simulink model "basic_model"  (R2024b)
settings: Solver=VariableStepAuto  StartTime=0.0  StopTime=0.4  FixedStep=5e-8  RelTol=1e-3

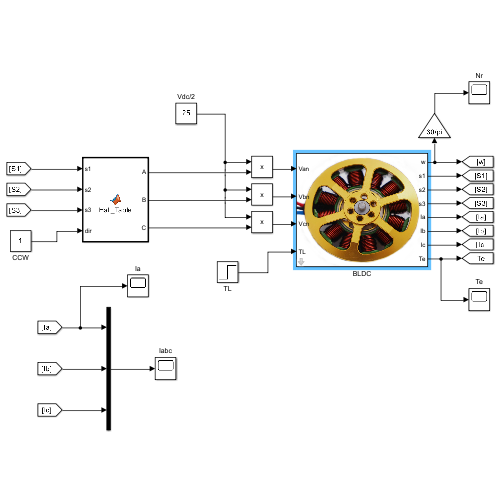
[thumbnail: Simulink's stored preview of the top-level diagram]
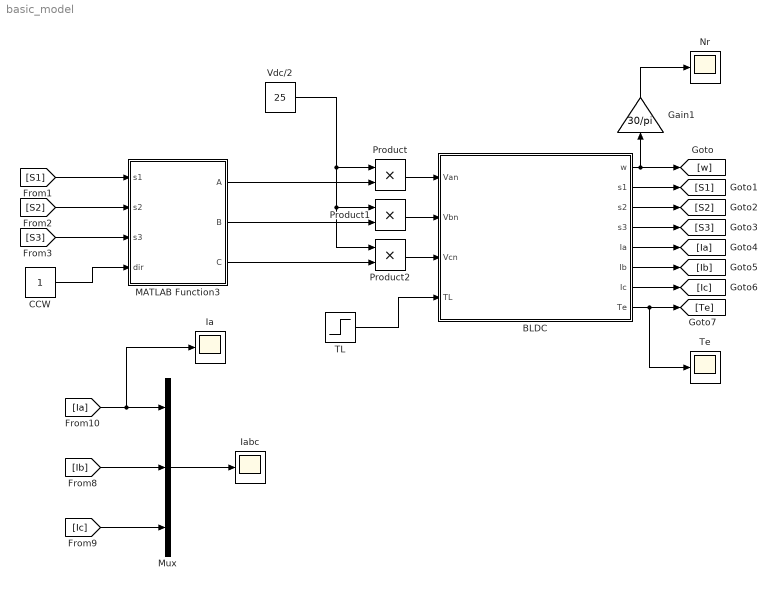
== system basic_model ==
  BLDC : Subsystem  mask(Function Block Parameters: BLDC){R=0.106/2, L=(0.428e-3)/2, b=0.0001, J=4.943e-4, Kt=0.164, Ke=0.164, pn=2}
      mask prompts: R "Phase Resistance"; L "Phase Inductance"; b "Viscous damping"; J "Rotor inertia"; Kt "Torque Sensitivity"; Ke "Back-EMF gain"; pn "poles pairs"
  CCW : Constant
  Gain1 : Gain  Gain=30/pi
  Ia : Scope
  Iabc : Scope
  MATLAB Function3 : MATLAB Function  TreatAsAtomicUnit=on
  Mux : Mux  Inputs=3
  Nr : Scope
  Product : Product
  Product1 : Product
  Product2 : Product
  TL : Step  Time=0.2  After=10  SampleTime=0
  Te : Scope
  Vdc/2 : Constant  Value=25
  wires:
  Vdc/2/1 -> Product2/1, Product1/1, Product/1
  BLDC/1(w) -> Gain1/1, [w]
  BLDC/2(s1) -> [S1]
  BLDC/3(s2) -> [S2]
  BLDC/4(s3) -> [S3]
  BLDC/5(Ia) -> [Ia]
  BLDC/6(Ib) -> [Ib]
  BLDC/7(Ic) -> [Ic]
  TL/1 -> BLDC/4(TL)
  [Ic] -> Mux/3
  [Ib] -> Mux/2
  [Ia] -> Ia/1, Mux/1
  MATLAB Function3/1(A) -> Product/2
  MATLAB Function3/2(B) -> Product1/2
  MATLAB Function3/3(C) -> Product2/2
  [S2] -> MATLAB Function3/2(s2)
  [S3] -> MATLAB Function3/3(s3)
  [S1] -> MATLAB Function3/1(s1)
  CCW/1 -> MATLAB Function3/4(dir)
  Gain1/1 -> Nr/1
  BLDC/8(Te) -> Te/1, [Te]
  Mux/1 -> Iabc/1
  Product2/1 -> BLDC/3(Vcn)
  Product/1 -> BLDC/1(Van)
  Product1/1 -> BLDC/2(Vbn)

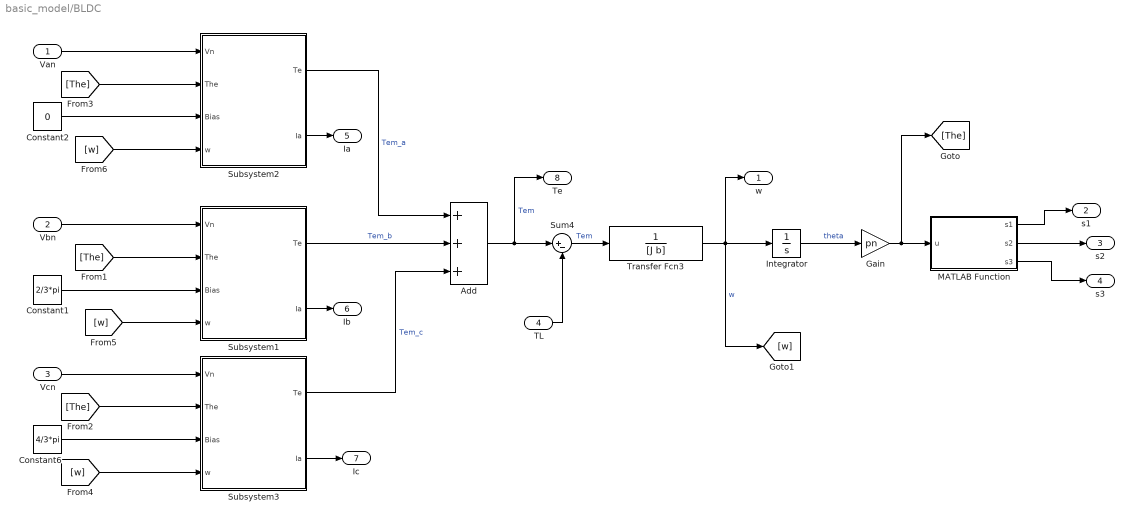
== system basic_model/BLDC ==
  Van : Inport
  Vbn : Inport  Port=2
  Vcn : Inport  Port=3
  TL : Inport  Port=4
  Add : Sum  Inputs=+++
  Constant1 : Constant  Value=2/3*pi
  Constant2 : Constant  Value=0
  Constant6 : Constant  Value=4/3*pi
  Gain : Gain  Gain=pn
  Integrator : Integrator
  MATLAB Function : MATLAB Function  TreatAsAtomicUnit=on
  Subsystem1 : Subsystem
  Subsystem2 : Subsystem
  Subsystem3 : Subsystem
  Sum4 : Sum  Inputs=|+-
  Transfer Fcn3 : TransferFcn  Denominator=[J b]
  w : Outport
  s1 : Outport  Port=2
  s2 : Outport  Port=3
  s3 : Outport  Port=4
  Ia : Outport  Port=5
  Ib : Outport  Port=6
  Ic : Outport  Port=7
  Te : Outport  Port=8
  wires:
  Vcn/1 -> Subsystem3/1(Vn)
  Sum4/1 -> Transfer Fcn3/1  "Tem"
  TL/1 -> Sum4/2
  Add/1 -> Te/1, Sum4/1  "Tem"
  Integrator/1 -> Gain/1  "theta"
  Transfer Fcn3/1 -> w/1, [w], Integrator/1  "w"
  [The] -> Subsystem3/2(The)
  Constant6/1 -> Subsystem3/3(Bias)
  Subsystem3/1(Te) -> Add/3  "Tem_c"
  Vbn/1 -> Subsystem1/1(Vn)
  Constant1/1 -> Subsystem1/3(Bias)
  [The] -> Subsystem1/2(The)
  Subsystem1/1(Te) -> Add/2  "Tem_b"
  Van/1 -> Subsystem2/1(Vn)
  Constant2/1 -> Subsystem2/3(Bias)
  [The] -> Subsystem2/2(The)
  Subsystem2/1(Te) -> Add/1  "Tem_a"
  [w] -> Subsystem3/4(w)
  [w] -> Subsystem1/4(w)
  [w] -> Subsystem2/4(w)
  Subsystem3/2(Ia) -> Ic/1
  Subsystem2/2(Ia) -> Ia/1
  MATLAB Function/1(s1) -> s1/1
  MATLAB Function/2(s2) -> s2/1
  MATLAB Function/3(s3) -> s3/1
  Subsystem1/2(Ia) -> Ib/1
  Gain/1 -> [The], MATLAB Function/1(u)

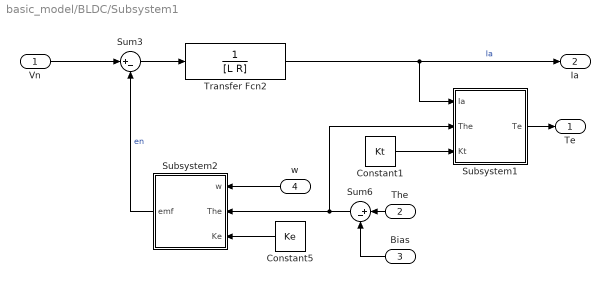
== system basic_model/BLDC/Subsystem1 ==
  Vn : Inport
  The : Inport  Port=2
  Bias : Inport  Port=3
  w : Inport  Port=4
  Constant1 : Constant  Value=Kt
  Constant5 : Constant  Value=Ke
  Subsystem1 : Subsystem
  Subsystem2 : Subsystem
  Sum3 : Sum  Inputs=|+-
  Sum6 : Sum  Inputs=|+-
  Transfer Fcn2 : TransferFcn  Denominator=[L R]
  Te : Outport
  Ia : Outport  Port=2
  wires:
  Bias/1 -> Sum6/2
  Subsystem2/1(emf) -> Sum3/2  "en"
  Sum6/1 -> Subsystem1/2(The), Subsystem2/2(The)
  Constant5/1 -> Subsystem2/3(Ke)
  w/1 -> Subsystem2/1(w)
  The/1 -> Sum6/1
  Constant1/1 -> Subsystem1/3(Kt)
  Subsystem1/1(Te) -> Te/1
  Sum3/1 -> Transfer Fcn2/1
  Vn/1 -> Sum3/1
  Transfer Fcn2/1 -> Subsystem1/1(Ia), Ia/1  "Ia"

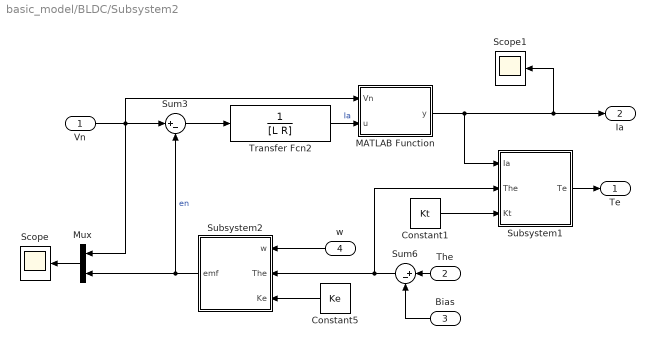
== system basic_model/BLDC/Subsystem2 ==
  Vn : Inport
  The : Inport  Port=2
  Bias : Inport  Port=3
  w : Inport  Port=4
  Constant1 : Constant  Value=Kt
  Constant5 : Constant  Value=Ke
  MATLAB Function : MATLAB Function  TreatAsAtomicUnit=on
  Mux : Mux  Inputs=2
  Scope : Scope
  Scope1 : Scope
  Subsystem1 : Subsystem
  Subsystem2 : Subsystem
  Sum3 : Sum  Inputs=|+-
  Sum6 : Sum  Inputs=|+-
  Transfer Fcn2 : TransferFcn  Denominator=[L R]
  Te : Outport
  Ia : Outport  Port=2
  wires:
  Bias/1 -> Sum6/2
  Subsystem2/1(emf) -> Sum3/2, Mux/2  "en"
  Sum6/1 -> Subsystem1/2(The), Subsystem2/2(The)
  Constant5/1 -> Subsystem2/3(Ke)
  w/1 -> Subsystem2/1(w)
  The/1 -> Sum6/1
  Constant1/1 -> Subsystem1/3(Kt)
  Subsystem1/1(Te) -> Te/1
  Mux/1 -> Scope/1
  Sum3/1 -> Transfer Fcn2/1
  Vn/1 -> Sum3/1, MATLAB Function/1(Vn), Mux/1
  Transfer Fcn2/1 -> MATLAB Function/2(u)  "Ia"
  MATLAB Function/1(y) -> Subsystem1/1(Ia), Scope1/1, Ia/1

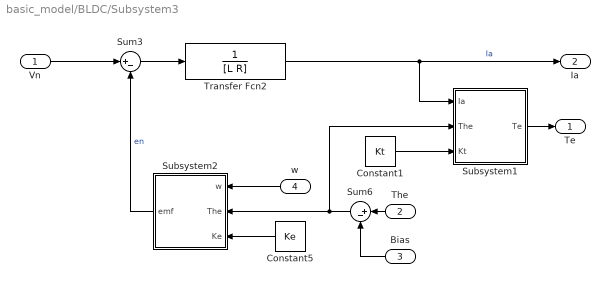
== system basic_model/BLDC/Subsystem3 ==
  Vn : Inport
  The : Inport  Port=2
  Bias : Inport  Port=3
  w : Inport  Port=4
  Constant1 : Constant  Value=Kt
  Constant5 : Constant  Value=Ke
  Subsystem1 : Subsystem
  Subsystem2 : Subsystem
  Sum3 : Sum  Inputs=|+-
  Sum6 : Sum  Inputs=|+-
  Transfer Fcn2 : TransferFcn  Denominator=[L R]
  Te : Outport
  Ia : Outport  Port=2
  wires:
  Bias/1 -> Sum6/2
  Subsystem2/1(emf) -> Sum3/2  "en"
  Sum6/1 -> Subsystem1/2(The), Subsystem2/2(The)
  Constant5/1 -> Subsystem2/3(Ke)
  w/1 -> Subsystem2/1(w)
  The/1 -> Sum6/1
  Constant1/1 -> Subsystem1/3(Kt)
  Subsystem1/1(Te) -> Te/1
  Sum3/1 -> Transfer Fcn2/1
  Vn/1 -> Sum3/1
  Transfer Fcn2/1 -> Subsystem1/1(Ia), Ia/1  "Ia"

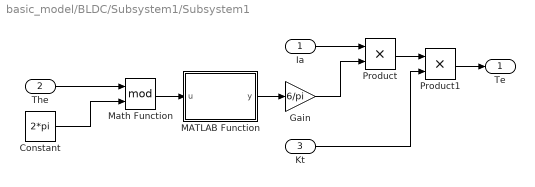
== system basic_model/BLDC/Subsystem1/Subsystem1 ==
  Ia : Inport
  The : Inport  Port=2
  Kt : Inport  Port=3
  Constant : Constant  Value=2*pi
  Gain : Gain  Gain=6/pi
  MATLAB Function : MATLAB Function  TreatAsAtomicUnit=on
  Math Function : Math  Operator=mod
  Product : Product
  Product1 : Product
  Te : Outport
  wires:
  The/1 -> Math Function/1
  Constant/1 -> Math Function/2
  Math Function/1 -> MATLAB Function/1(u)
  MATLAB Function/1(y) -> Gain/1
  Ia/1 -> Product/1
  Gain/1 -> Product/2
  Product/1 -> Product1/1
  Kt/1 -> Product1/2
  Product1/1 -> Te/1

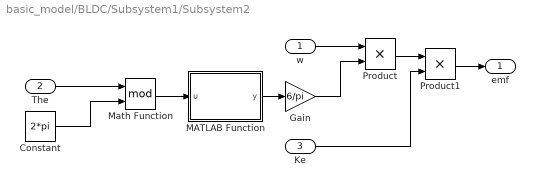
== system basic_model/BLDC/Subsystem1/Subsystem2 ==
  w : Inport
  The : Inport  Port=2
  Ke : Inport  Port=3
  Constant : Constant  Value=2*pi
  Gain : Gain  Gain=6/pi
  MATLAB Function : MATLAB Function  TreatAsAtomicUnit=on
  Math Function : Math  Operator=mod
  Product : Product
  Product1 : Product
  emf : Outport
  wires:
  The/1 -> Math Function/1
  Constant/1 -> Math Function/2
  Math Function/1 -> MATLAB Function/1(u)
  MATLAB Function/1(y) -> Gain/1
  w/1 -> Product/1
  Gain/1 -> Product/2
  Product/1 -> Product1/1
  Ke/1 -> Product1/2
  Product1/1 -> emf/1

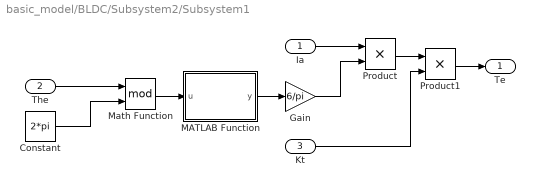
== system basic_model/BLDC/Subsystem2/Subsystem1 ==
  Ia : Inport
  The : Inport  Port=2
  Kt : Inport  Port=3
  Constant : Constant  Value=2*pi
  Gain : Gain  Gain=6/pi
  MATLAB Function : MATLAB Function  TreatAsAtomicUnit=on
  Math Function : Math  Operator=mod
  Product : Product
  Product1 : Product
  Te : Outport
  wires:
  The/1 -> Math Function/1
  Constant/1 -> Math Function/2
  Math Function/1 -> MATLAB Function/1(u)
  MATLAB Function/1(y) -> Gain/1
  Ia/1 -> Product/1
  Gain/1 -> Product/2
  Product/1 -> Product1/1
  Kt/1 -> Product1/2
  Product1/1 -> Te/1

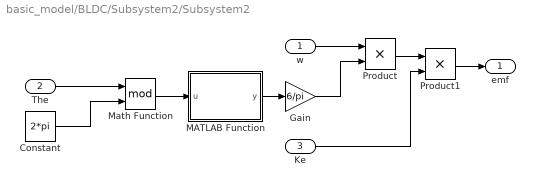
== system basic_model/BLDC/Subsystem2/Subsystem2 ==
  w : Inport
  The : Inport  Port=2
  Ke : Inport  Port=3
  Constant : Constant  Value=2*pi
  Gain : Gain  Gain=6/pi
  MATLAB Function : MATLAB Function  TreatAsAtomicUnit=on
  Math Function : Math  Operator=mod
  Product : Product
  Product1 : Product
  emf : Outport
  wires:
  The/1 -> Math Function/1
  Constant/1 -> Math Function/2
  Math Function/1 -> MATLAB Function/1(u)
  MATLAB Function/1(y) -> Gain/1
  w/1 -> Product/1
  Gain/1 -> Product/2
  Product/1 -> Product1/1
  Ke/1 -> Product1/2
  Product1/1 -> emf/1

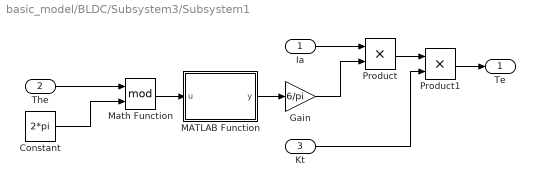
== system basic_model/BLDC/Subsystem3/Subsystem1 ==
  Ia : Inport
  The : Inport  Port=2
  Kt : Inport  Port=3
  Constant : Constant  Value=2*pi
  Gain : Gain  Gain=6/pi
  MATLAB Function : MATLAB Function  TreatAsAtomicUnit=on
  Math Function : Math  Operator=mod
  Product : Product
  Product1 : Product
  Te : Outport
  wires:
  The/1 -> Math Function/1
  Constant/1 -> Math Function/2
  Math Function/1 -> MATLAB Function/1(u)
  MATLAB Function/1(y) -> Gain/1
  Ia/1 -> Product/1
  Gain/1 -> Product/2
  Product/1 -> Product1/1
  Kt/1 -> Product1/2
  Product1/1 -> Te/1

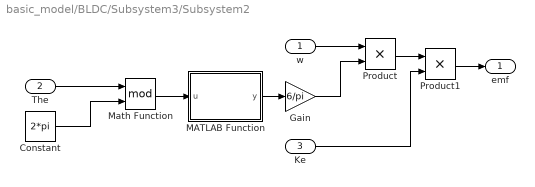
== system basic_model/BLDC/Subsystem3/Subsystem2 ==
  w : Inport
  The : Inport  Port=2
  Ke : Inport  Port=3
  Constant : Constant  Value=2*pi
  Gain : Gain  Gain=6/pi
  MATLAB Function : MATLAB Function  TreatAsAtomicUnit=on
  Math Function : Math  Operator=mod
  Product : Product
  Product1 : Product
  emf : Outport
  wires:
  The/1 -> Math Function/1
  Constant/1 -> Math Function/2
  Math Function/1 -> MATLAB Function/1(u)
  MATLAB Function/1(y) -> Gain/1
  w/1 -> Product/1
  Gain/1 -> Product/2
  Product/1 -> Product1/1
  Ke/1 -> Product1/2
  Product1/1 -> emf/1

== matlab function basic_model/BLDC/Subsystem1/Subsystem1/MATLAB Function ==
function y = The_t(u)
if u <= pi/6
    y = u;
elseif u < 5/6*pi
    y = pi/6;
elseif u < 7/6*pi
    y = pi - u;
elseif u < 11/6*pi
    y = -pi/6;
else 
    y = u - 2*pi;
end

== matlab function basic_model/BLDC/Subsystem1/Subsystem2/MATLAB Function ==
function y = The_t(u)
if u <= pi/6
    y = u;
elseif u < 5/6*pi
    y = pi/6;
elseif u < 7/6*pi
    y = pi - u;
elseif u < 11/6*pi
    y = -pi/6;
else 
    y = u - 2*pi;
end

== matlab function basic_model/BLDC/Subsystem2/Subsystem1/MATLAB Function ==
function y = The_t(u)
if u <= pi/6
    y = u;
elseif u < 5/6*pi
    y = pi/6;
elseif u < 7/6*pi
    y = pi - u;
elseif u < 11/6*pi
    y = -pi/6;
else 
    y = u - 2*pi;
end

== matlab function basic_model/BLDC/Subsystem3/Subsystem1/MATLAB Function ==
function y = The_t(u)
if u <= pi/6
    y = u;
elseif u < 5/6*pi
    y = pi/6;
elseif u < 7/6*pi
    y = pi - u;
elseif u < 11/6*pi
    y = -pi/6;
else 
    y = u - 2*pi;
end

== matlab function basic_model/BLDC/Subsystem3/Subsystem2/MATLAB Function ==
function y = The_t(u)
if u <= pi/6
    y = u;
elseif u < 5/6*pi
    y = pi/6;
elseif u < 7/6*pi
    y = pi - u;
elseif u < 11/6*pi
    y = -pi/6;
else 
    y = u - 2*pi;
end

== matlab function basic_model/BLDC/Subsystem2/Subsystem2/MATLAB Function ==
function y = The_t(u)
if u <= pi/6
    y = u;
elseif u < 5/6*pi
    y = pi/6;
elseif u < 7/6*pi
    y = pi - u;
elseif u < 11/6*pi
    y = -pi/6;
else 
    y = u - 2*pi;
end

== matlab function basic_model/BLDC/MATLAB Function ==
function [s1,s2,s3] = Hall_sensor(u)
    u = mod((u - pi/6),2*pi);
    sector = fix(u/(pi/3)) + 1;
    if sector > 6
        sector = 1;
    end
    Hall_Tab = [1 0 1;1 0 0;1 1 0;0 1 0; 0 1 1;0 0 1];
    s1 = Hall_Tab(sector,1);
    s2 = Hall_Tab(sector,2);
    s3 = Hall_Tab(sector,3);
end

== matlab function basic_model/BLDC/Subsystem2/MATLAB Function ==
function y = fcn(Vn,u)
if Vn == 0
    u = 0;
end
y = u;

== matlab function basic_model/MATLAB Function3 ==
function [A,B,C] = Hall_Table(s1,s2,s3,dir)
    states = s1*4 + s2*2 + s3*1;
    if states == 0 || states == 7
        A = 0;
        B = 0;
        C = 0; % error Hall signals, stop motor
        return;
    end
    %map table
    map_tab = [6, 4, 5, 2, 1, 3];
    six_commut_tab = [1,-1,0; 1,0,-1;0,1,-1;-1,1,0;-1,0,1;0,-1,1];
    if dir > 0 %CCW, forward rotation
        index = map_tab(states);
    else %CW, reversal rotation
        index = mod(map_tab(states) - 1 + 3,6) + 1;
    end
    A = six_commut_tab(index,1);
    B = six_commut_tab(index,2);
    C = six_commut_tab(index,3);
end
